simulink model "WIP_1g"  (R2025b)
settings: Solver=ode15s  StartTime=0.0  StopTime=10  MaxStep=1e-2  RelTol=1e-5
InitFcn:
  | run("init.m");
settings Model: Creator=Acer  LastModifiedBy=Acer
settings SolverCC: InitialStep=1e-5  SolverResetMethod=Robust

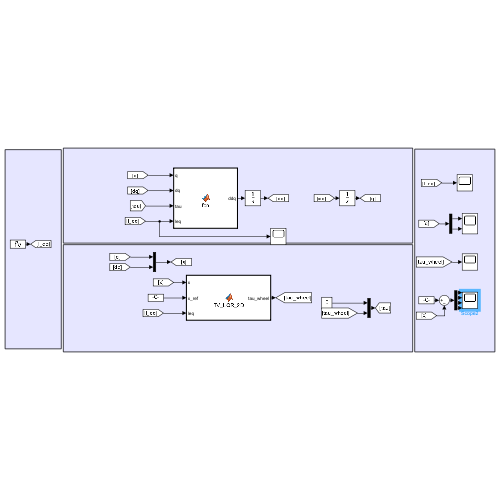
[thumbnail: Simulink's stored preview of the top-level diagram]
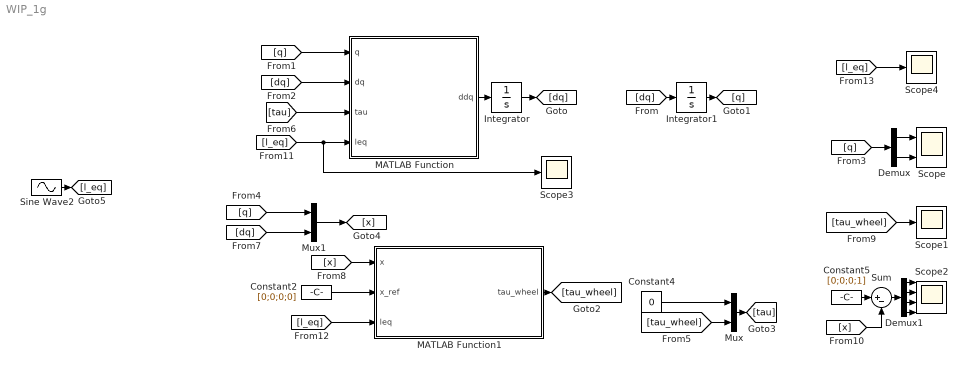
== system WIP_1g ==
  Constant2 : Constant  Value=[0;0;0;0]
  Constant4 : Constant  Value=0
  Constant5 : Constant  Value=[0;0;0;1]
  Demux : Demux  Outputs=2
  Demux1 : Demux
  Integrator : Integrator  InitialCondition=[0;0]  ContinuousStateAttributes="\"dq\""
  Integrator1 : Integrator  InitialCondition=[0.01;0]  ContinuousStateAttributes="\"q\""
  MATLAB Function : MATLAB Function  TreatAsAtomicUnit=on
  MATLAB Function1 : MATLAB Function  TreatAsAtomicUnit=on
  Mux : Mux  Inputs=2
  Mux1 : Mux  Inputs=2
  Scope : Scope  NumInputPorts=2
      settings: Title=qw  ActiveDisplayYMinimum=-0.025741465119678165  ActiveDisplayYMaximum=0.23167318607710355
  Scope1 : Scope
      settings: ActiveDisplayYMinimum=3.5772245612537574  ActiveDisplayYMaximum=23.577224561253757
  Scope2 : Scope  NumInputPorts=4
      settings: ActiveDisplayString=4  Title=dqw  ActiveDisplayYMinimum=0.30680092618848021  ActiveDisplayYMaximum=1.160527473131344  DataLoggingVariableName=ScopeData2
  Scope3 : Scope
      settings: ActiveDisplayYMinimum=0.77592818295080312  ActiveDisplayYMaximum=1.0248968685610218  DataLoggingVariableName=ScopeData3
  Scope4 : Scope
      settings: ActiveDisplayYMinimum=0.77500000154560889  ActiveDisplayYMaximum=1.0249999998282657  DataLoggingVariableName=ScopeData4
  Sine Wave2 : Sin  Amplitude=.1  Bias=0.9  Frequency=2  Phase=pi/2  SampleTime=0
  Sum : Sum  Inputs=|+-
  wires:
  MATLAB Function/1(ddq) -> Integrator/1
  Integrator/1 -> [dq]
  [dq] -> Integrator1/1
  Integrator1/1 -> [q]
  [q] -> MATLAB Function/1(q)
  [dq] -> MATLAB Function/2(dq)
  [l_eq] -> Scope3/1, MATLAB Function/4(leq)
  Demux/1 -> Scope/1
  [q] -> Demux/1
  Demux/2 -> Scope/2
  Constant2/1 -> MATLAB Function1/2(x_ref)
  [l_eq] -> MATLAB Function1/3(leq)
  MATLAB Function1/1(tau_wheel) -> [tau_wheel]
  [tau_wheel] -> Mux/2
  Constant4/1 -> Mux/1
  Mux/1 -> [tau]
  [tau] -> MATLAB Function/3(tau)
  [q] -> Mux1/1
  [dq] -> Mux1/2
  Mux1/1 -> [x]
  [x] -> MATLAB Function1/1(x)
  [tau_wheel] -> Scope1/1
  [x] -> Sum/2
  Constant5/1 -> Sum/1
  Sum/1 -> Demux1/1
  Demux1/1 -> Scope2/1
  Demux1/2 -> Scope2/2
  Demux1/3 -> Scope2/3
  Demux1/4 -> Scope2/4
  Sine Wave2/1 -> [l_eq]
  [l_eq] -> Scope4/1

== matlab function WIP_1g/MATLAB Function1 ==
  data: x input double size=4; tau_wheel output; x_ref input double size=4; leq input double size=1; robot_params parameter
function tau_wheel = TV_LQR_2D(x, x_ref, leq, robot_params)
    % x: Stato attuale [s; theta; phi; s_dot; theta_dot; phi_dot] (6x1)
    % x_ref: Stato target desiderato [s_ref; theta_ref; phi_ref; 0; 0; 0] (6x1)
    % l: Lunghezza attuale del pendolo equivalente [m]
    % I_y: Inerzia attuale del corpo superiore [kg*m^2]
    
    coder.extrinsic('lqr');

    m_eq = robot_params.meq;
    mw = robot_params.mw;
    Rw = robot_params.Rw;
    Iw= robot_params.Iw;
    g = robot_params.g;
    bw =  robot_params.bw;
    
    % Evita divisioni per zero al primo step di simulazione
    if leq < 1e-4
        leq = 1e-4;
    end
    
    A = [0, 0, 1,0;
         0, 0, 0,1;
        (g*(Iw + Rw^2*m_eq + Rw^2*mw))/(leq*(mw*Rw^2 + Iw)), 0, 0, (Rw*bw)/(leq*(mw*Rw^2 + Iw));
        -(Rw*g*m_eq)/(mw*Rw^2 + Iw), 0, 0,           -bw/(mw*Rw^2 + Iw)];
 
    B = [0;0;-Rw/(leq*(mw*Rw^2 + Iw));1/(mw*Rw^2 + Iw)];

    %x = [q1, qw,  dot_qw,  dot_q1]
    % U = [tau_wheel]
    Q = diag([200,10,10, 10]);
    R = 0.01;         % uso coppie piu abbasso piu accelera
    
    % 5. Risoluzione LQR e Calcolo Input
    % Inizializza K per la Code Generation di Simulink
    K = zeros(1, 4); 
    
    % Calcola la matrice dei guadagni ottimali K
    K = lqr(A, B, Q, R);
    
    % Errore di stato (tilde_X)
    X_tilde = x - x_ref;
    
    tau_wheel = -K * X_tilde; 
end

== matlab function WIP_1g/MATLAB Function ==
  settings: updateMethod=CONTINUOUS
  data: q input double size=2; dq input double size=2; tau input; leq input; ddq output double size=2; robot_params parameter
function ddq = fcn(q,dq,tau, leq,robot_params)


q1 = q(1);
qw = q(2);

dq1 = dq(1);
dqw = dq(2);

m_eq = robot_params.meq;
mw = robot_params.mw;
Rw = robot_params.Rw;
Iw= robot_params.Iw;
g = robot_params.g;
bw =  robot_params.bw;

M = [ m_eq.*leq.^2 , m_eq.*Rw*leq*cos(q1);
     m_eq.*Rw.*leq.*cos(q1) , (m_eq + mw).*Rw.^2+Iw];

 C = [0, 0;
     -Rw*dq1*leq*m_eq*sin(q1), bw];

G = [-m_eq.*g.*leq.*sin(q1);0];

ddq = M\(-C*dq -G + tau);
